simulink model "PSC_DynoLoadTorque"  (R2022b)
settings: Solver=FixedStepDiscrete  StartTime=0.0  StopTime=SimTime  FixedStep=Ts_Model  RelTol=1e-3
settings Model: Creator=BEDNASA  LastModifiedBy=HENRIE2
settings SolverCC: AlgebraicLoopSolver=TrustRegion
settings DebuggingCC: UnconnectedInputMsg=warning  UnconnectedOutputMsg=warning  UnconnectedLineMsg=warning  SFMachineParentedDataDiag=warning
settings ModelReferenceCC: EnableRefExpFcnMdlSchedulingChecks=on  ModelReferenceNumInstancesAllowed=Single
settings RTWCC: CustomInclude="\"C:\\Users\\BEDNASA\\Desktop\\VA_PSCSimulationArchitecture (2)\\VA_PSCSimulationArchitecture\\tools\\FMIKit-Simulink-2.7\\include\" \"C:\\Users\\BEDNASA\\Desktop\\SPPMSM\\SPPMSM\\SinglePhaseSimArch_alpha\\tools\\FMIKit-Simulink-2.8\\include\" \"C:\\Users\\BEDNASA\\Desktop\\SPPMSM\\SPPMSM\\MBD_SPM_SimArch\\tools\\include\" \"C:\\Users\\BEDNASA\\Desktop\\SPPMSM\\SPPMSM\\MBD_SPM_SimArch\\tools\\FMIKit\\FMIKit-Simulink-2.9\\include\" \"C:\\Data\\MBD_SPM_SimArch\\tools\\FMIKit\\FMIKit-Simulink-2.9\\include\""  CustomSource="\"C:\\Users\\BEDNASA\\Desktop\\VA_PSCSimulationArchitecture (2)\\VA_PSCSimulationArchitecture\\tools\\FMIKit-Simulink-2.7\\src\\FMU.cpp\" \"C:\\Users\\BEDNASA\\Desktop\\VA_PSCSimulationArchitecture (2)\\VA_PSCSimulationArchitecture\\tools\\FMIKit-Simulink-2.7\\src\\FMU1.cpp\" \"C:\\Users\\BEDNASA\\Desktop\\VA_PSCSimulationArchitecture (2)\\VA_PSCSimulationArchitecture\\tools\\FMIKit-Simulink-2.7\\src\\FMU2.cpp\" \"C:\\Users\\BEDNASA\\Desktop\\SPPMSM\\SPPMSM\\SinglePhaseSimArch_alpha\\tools\\FMIKit-Simulink-2.8\\src\\FMU.cpp\" \"C:\\Users\\BEDNASA\\Desktop\\SPPMSM\\SPPMSM\\SinglePhaseSimArch_alpha\\tools\\FMIKit-Simulink-2.8\\src\\FMU1.cpp\" \"C:\\Users\\BEDNASA\\Desktop\\SPPMSM\\SPPMSM\\SinglePhaseSimArch_alpha\\tools\\FMIKit-Simulink-2.8\\src\\FMU2.cpp\" \"C:\\Users\\BEDNASA\\Desktop\\SPPMSM\\SPPMSM\\MBD_SPM_SimArch\\tools\\src\\FMU.cpp\" \"C:\\Users\\BEDNASA\\Desktop\\SPPMSM\\SPPMSM\\MBD_SPM_SimArch\\tools\\src\\FMU1.cpp\" \"C:\\Users\\BEDNASA\\Desktop\\SPPMSM\\SPPMSM\\MBD_SPM_SimArch\\tools\\src\\FMU2.cpp\" \"C:\\Users\\BEDNASA\\Desktop\\SPPMSM\\SPPMSM\\MBD_SPM_SimArch\\tools\\FMIKit\\FMIKit-Simulink-2.9\\src\\FMU.cpp\" \"C:\\Users\\BEDNASA\\Desktop\\SPPMSM\\SPPMSM\\MBD_SPM_SimArch\\tools\\FMIKit\\FMIKit-Simulink-2.9\\src\\FMU1.cpp\" \"C:\\Users\\BEDNASA\\Desktop\\SPPMSM\\SPPMSM\\MBD_SPM_SimArch\\tools\\FMIKit\\FMIKit-Simulink-2.9\\src\\FMU2.cpp\" \"C:\\Data\\MBD_SPM_SimArch\\tools\\FMIKit\\FMIKit-Simulink-2.9\\src\\FMU.cpp\" \"C:\\Data\\MBD_SPM_SimArch\\tools\\FMIKit\\FMIKit-Simulink-2.9\\src\\FMU1.cpp\" \"C:\\Data\\MBD_SPM_SimArch\\tools\\FMIKit\\FMIKit-Simulink-2.9\\src\\FMU2.cpp\""  CustomLibrary="\"C:\\Program Files\\Microsoft SDKs\\Windows\\v6.0A\\Lib\\x64\\ShLwApi.Lib\""

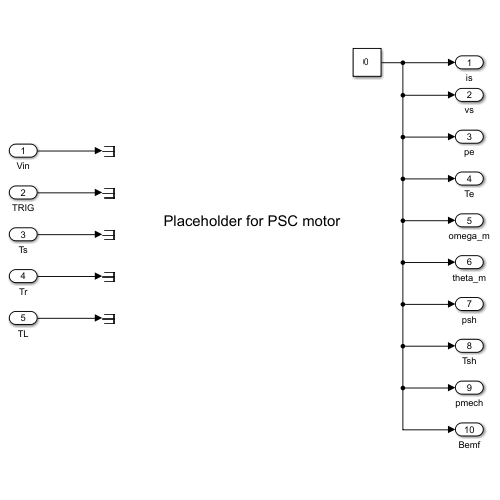
[thumbnail: Simulink's stored preview of the top-level diagram]
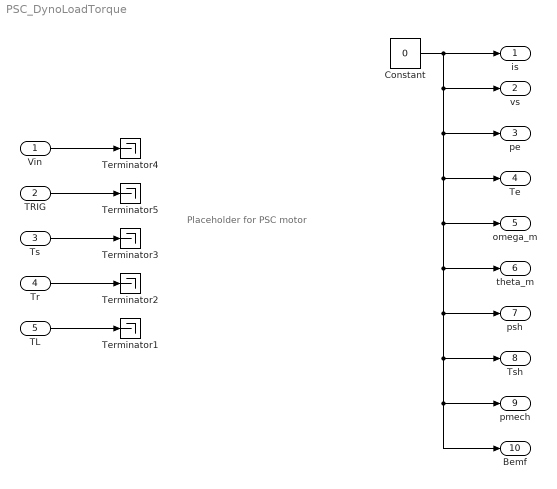
== system PSC_DynoLoadTorque ==
  note: Placeholder for PSC motor
  Vin : Inport
  TRIG : Inport  Port=2
  Ts : Inport  Port=3
  Tr : Inport  Port=4
  TL : Inport  Port=5
  Constant : Constant  Value=0
  Terminator{1..5} (5 alike) : Terminator
  is : Outport
  vs : Outport  Port=2
  pe : Outport  Port=3
  Te : Outport  Port=4
  omega_m : Outport  Port=5
  theta_m : Outport  Port=6
  psh : Outport  Port=7
  Tsh : Outport  Port=8
  pmech : Outport  Port=9
  Bemf : Outport  Port=10
  wires:
  Ts/1 -> Terminator3/1
  Tr/1 -> Terminator2/1
  TRIG/1 -> Terminator5/1
  TL/1 -> Terminator1/1
  Vin/1 -> Terminator4/1
  Constant/1 -> Bemf/1, pmech/1, Tsh/1, psh/1, theta_m/1, omega_m/1, Te/1, pe/1, vs/1, is/1
